simulink model "VCMGCM1962020b_v2"  (R2020b)
settings: Solver=FixedStepDiscrete  StartTime=0.0  StopTime=10.0  FixedStep=0.005  RelTol=1e-3  EnableMultiTasking=on
PreLoadFcn:
  | try, model_open; catch, disp('Error occurred while executing model pre-load callback: model_open.m'); disp('Please assure that the MATLAB working directory is set to the model directory before opening.'); end
InitFcn:
  | try, model_open; catch, end
undefined symbols (not defined in the file): Bridge, GCM, H, raptor_get_param_eval, raptor_get_safe_string, raptor_xcp_function
libraries: Blocks_lib x1165, Raptor_lib x665, simulink x62, VCM_lib x5
(part 16 of 23)

== system VCMGCM1962020b_v2/Fgnd/Actuators/CAN/Display/DisplayHVES1_D2/MsgTx ==
  Data : Inport
  Enable : EnablePort
  Bus Selector1 : BusSelector  OutputSignals=VirtualSensors.Batt.BattSOC [%]
  Bus Selector2 : BusSelector  OutputSignals=Sensors.CAN.Other.BCM.CCVS1_BCM.Parking_Brak_Switch.Parking_Brak_Switch [enum],VirtualSensors.Spd.VehSpd [kph]
  Bus Selector3 : BusSelector  OutputSignals=Sensors.CAN.Other.BCM.BCMAMB.Amb_Air_Temp.Amb_Air_Temp [C]
  Bus Selector4 : BusSelector  OutputSignals=VirtualSensors.Spd.VehOdmtr [km],VirtualSensors.Spd.TripDist [km]
  Bus Selector5 : BusSelector  OutputSignals=VirtualSensors.Batt.BattCur [A],VirtualSensors.Batt.BattVolt [V]
  Bus Selector6 : BusSelector  OutputSignals=Control.Other.Other.Regenstate
  Bus Selector7 : BusSelector  OutputSignals=Control.Mode.StartStop.ChgMode [Bool]
  Bus Selector8 : BusSelector  OutputSignals=VirtualSensors.Spd.VehRangeEst [km]
  Bus Selector9 : BusSelector  OutputSignals=Control.Mode.PRNDMode_Act [enum]
  CANTxField{,4..6,8..10} (7 alike) : Blocks_lib/CANTxField  Commented=on  custom=on  custom_nam=[nam '---']  custom_units='---'
  CANTxField{1..3,7} (4 alike) : Blocks_lib/CANTxField  custom=on  custom_nam=[nam '---']  custom_units='---'
  Header : Blocks_lib/Header  width=Landscape  addtext=''
  raptor_can_txmsg : Raptor_lib/CAN/raptor_can_txmsg  Commented=on  canDefinition=struct('dbcFile', 'Drivers_Disp_dbc_file_v5.0.dbc','message', 'CCVS1','comment', '','signals', {{'P_Brake_Switch','Whl_Veh_Spd'}},'enabled', [ 1 1;],'scaled', [ 1 1;],'canBus', 'bus','messageID', [ 419361263;],'idMask', [ 536870911;],'payloadMask', [],'payloadValue', [],'period', [ 100;],'mailbox', '''''','queueSize', [ 1;],'label', [ 1;],'ver', [ 2;],'showID', [ 0;],'showRaw', [ 0;],'fill', [ 0;],'editID', [ 0;],'signalOrder', [ 1;],'signalAscDes', [ 1;])  canBus=bus  queueSize=1  payloadMask=[]  payloadValue=[]  period=100  showID=0  label=1  idMask=hex2dec('1FFFFFFF')  fill=0  id=419361263  showRaw=0  signalOrder=1  signalInfo={{struct('Name', 'Whl_Veh_Spd','Startbit', [ 0;],'SignalSize', [ 16;],'ByteOrder', 'LittleEndian','ValueType', 'UNSIGNED','Class', 'uint16','Signed', [ 0;],'Factor', [ 0.0039063;],'Offset', [ 0;],'Min', [ 0;],'Max', [ 250.996;],'Units', 'Km/h','Comment', '','StartBit', [ 8;]),struct('Name', 'P_Brake_Switch','Startbit', [ 0;],'SignalSize', [ 2;],'ByteOrder', 'LittleEndian','ValueType', 'UNSIGNED','Class', 'uint8','Signed', [ 0;],'Factor', [ 1;],'Offset', [ 0;],'Min', [ 0;],'Max', [ 3;],'Units', 'enum','Comment', '','StartBit', [ 2;])}}
      settings: SourceProductName=Raptor
  raptor_can_txmsg1 : Raptor_lib/CAN/raptor_can_txmsg  canDefinition=struct('dbcFile', 'Drivers_Disp_dbc_file_v5.0.dbc','message', 'HVES1_D2','comment', '','signals', {{'Batt_SOC'}},'enabled', [ 1;],'scaled', [ 1;],'canBus', 'bus','messageID', [ 418419183;],'idMask', [ 536870911;],'payloadMask', [],'payloadValue', [],'period', [ 100;],'mailbox', '''''','queueSize', [ 1;],'label', [ 1;],'ver', [ 2;],'showID', [ 0;],'showRaw', [ 0;],'fill', [ 0;],'editID', [ 0;],'signalOrder', [ 1;],'signalAscDes', [ 1;])  canBus=bus  queueSize=1  payloadMask=[]  payloadValue=[]  period=100  showID=0  label=1  idMask=hex2dec('1FFFFFFF')  fill=0  id=418419183  showRaw=0  signalOrder=1  signalInfo={{struct('Name', 'Batt_SOC','Startbit', [ 0;],'SignalSize', [ 16;],'ByteOrder', 'LittleEndian','ValueType', 'UNSIGNED','Class', 'uint16','Signed', [ 0;],'Factor', [ 0.0015625;],'Offset', [ 0;],'Min', [ 0;],'Max', [ 100.398;],'Units', '%','Comment', '','StartBit', [ 0;])}}
      settings: SourceProductName=Raptor
  raptor_can_txmsg2 : Raptor_lib/CAN/raptor_can_txmsg  Commented=on  canDefinition=struct('dbcFile', 'Drivers_Disp_dbc_file_v5.0.dbc','message', 'AMB','comment', '','signals', {{'Ambient_Air_Temperature','Cab_Temp'}},'enabled', [ 1 0;],'scaled', [ 1 1;],'canBus', 'bus','messageID', [ 419362081;],'idMask', [ 536870911;],'payloadMask', [],'payloadValue', [],'period', [ 100;],'mailbox', '''''','queueSize', [ 1;],'label', [ 1;],'ver', [ 2;],'showID', [ 0;],'showRaw', [ 0;],'fill', [ 0;],'editID', [ 0;],'signalOrder', [ 1;],'signalAscDes', [ 1;])  canBus=bus  queueSize=1  payloadMask=[]  payloadValue=[]  period=100  showID=0  label=1  idMask=hex2dec('1FFFFFFF')  fill=0  id=419362081  showRaw=0  signalOrder=1  signalInfo={{struct('Name', 'Ambient_Air_Temperature','Startbit', [ 0;],'SignalSize', [ 16;],'ByteOrder', 'LittleEndian','ValueType', 'UNSIGNED','Class', 'uint16','Signed', [ 0;],'Factor', [ 0.03125;],'Offset', [ -22;],'Min', [ -22;],'Max', [ 140;],'Units', 'C','Comment', '','StartBit', [ 24;]),struct('Name', 'Cab_Temp','Startbit', [ 0;],'SignalSize', [ 16;],'ByteOrder', 'LittleEndian','ValueType', 'UNSIGNED','Class', 'uint16','Signed', [ 0;],'Factor', [ 0.03125;],'Offset', [ -22;],'Min', [ -22;],'Max', [ 140;],'Units', 'C','Comment', '','StartBit', [ 8;])}}
      settings: SourceProductName=Raptor
  raptor_can_txmsg3 : Raptor_lib/CAN/raptor_can_txmsg  canDefinition=struct('dbcFile', 'Drivers_Disp_dbc_file_v5.0.dbc','message', 'OI','comment', '','signals', {{'Range_Estimate'}},'enabled', [ 1;],'scaled', [ 1;],'canBus', 'bus','messageID', [ 419364847;],'idMask', [ 536870911;],'payloadMask', [],'payloadValue', [],'period', [ 100;],'mailbox', '''''','queueSize', [ 1;],'label', [ 1;],'ver', [ 2;],'showID', [ 0;],'showRaw', [ 0;],'fill', [ 0;],'editID', [ 0;],'signalOrder', [ 1;],'signalAscDes', [ 1;])  canBus=bus  queueSize=1  payloadMask=[]  payloadValue=[]  period=100  showID=0  label=1  idMask=hex2dec('1FFFFFFF')  fill=0  id=419364847  showRaw=0  signalOrder=1  signalInfo={{struct('Name', 'Range_Estimate','Startbit', [ 0;],'SignalSize', [ 16;],'ByteOrder', 'LittleEndian','ValueType', 'UNSIGNED','Class', 'uint16','Signed', [ 0;],'Factor', [ 1;],'Offset', [ 0;],'Min', [ 0;],'Max', [ 64255;],'Units', 'km','Comment', '','StartBit', [ 16;])}}
      settings: SourceProductName=Raptor
  raptor_can_txmsg4 : Raptor_lib/CAN/raptor_can_txmsg  canDefinition=struct('dbcFile', 'Drivers_Disp_dbc_file_v5.0.dbc','message', 'VDHR','comment', '','signals', {{'Tot_Veh_Dist','Trip_Dist'}},'enabled', [ 1 1;],'scaled', [ 1 1;],'canBus', 'bus','messageID', [ 419348975;],'idMask', [ 536870911;],'payloadMask', [],'payloadValue', [],'period', [ 100;],'mailbox', '''''','queueSize', [ 1;],'label', [ 1;],'ver', [ 2;],'showID', [ 0;],'showRaw', [ 0;],'fill', [ 0;],'editID', [ 0;],'signalOrder', [ 1;],'signalAscDes', [ 1;])  canBus=bus  queueSize=1  payloadMask=[]  payloadValue=[]  period=100  showID=0  label=1  idMask=hex2dec('1FFFFFFF')  fill=0  id=419348975  showRaw=0  signalOrder=1  signalInfo={{struct('Name', 'Tot_Veh_Dist','Startbit', [ 0;],'SignalSize', [ 32;],'ByteOrder', 'LittleEndian','ValueType', 'UNSIGNED','Class', 'uint32','Signed', [ 0;],'Factor', [ 5;],'Offset', [ 0;],'Min', [ 0;],'Max', [ 419436000;],'Units', 'm','Comment', '','StartBit', [ 0;]),struct('Name', 'Trip_Dist','Startbit', [ 0;],'SignalSize', [ 32;],'ByteOrder', 'LittleEndian','ValueType', 'UNSIGNED','Class', 'uint32','Signed', [ 0;],'Factor', [ 5;],'Offset', [ 0;],'Min', [ 0;],'Max', [ 419436000;],'Units', 'm','Comment', '','StartBit', [ 32;])}}
      settings: SourceProductName=Raptor
  raptor_can_txmsg5 : Raptor_lib/CAN/raptor_can_txmsg  Commented=on  canDefinition=struct('dbcFile', 'Drivers_Disp_dbc_file_v3.dbc','message', 'HVES1_D1','comment', '','signals', {{'Batt_Current','Batt_Voltage_Level'}},'enabled', [ 1 1;],'scaled', [ 1 1;],'canBus', 'bus','messageID', [ 217092335;],'idMask', [ 536870911;],'payloadMask', [],'payloadValue', [],'period', [ 100;],'mailbox', '''''','queueSize', [ 1;],'label', [ 1;],'ver', [ 2;],'showID', [ 0;],'showRaw', [ 0;],'fill', [ 0;],'editID', [ 0;],'signalOrder', [ 1;],'signalAscDes', [ 1;])  canBus=bus  queueSize=1  payloadMask=[]  payloadValue=[]  period=100  showID=0  label=1  idMask=hex2dec('1FFFFFFF')  fill=0  id=217092335  showRaw=0  signalOrder=1  signalInfo={{struct('Name', 'Batt_Voltage_Level','Startbit', [ 0;],'SignalSize', [ 16;],'ByteOrder', 'LittleEndian','ValueType', 'UNSIGNED','Class', 'uint16','Signed', [ 0;],'Factor', [ 0.05;],'Offset', [ 0;],'Min', [ 0;],'Max', [ 3212.75;],'Units', 'V','Comment', '','StartBit', [ 32;]),struct('Name', 'Batt_Current','Startbit', [ 0;],'SignalSize', [ 16;],'ByteOrder', 'LittleEndian','ValueType', 'UNSIGNED','Class', 'uint16','Signed', [ 0;],'Factor', [ 0.05;],'Offset', [ -1600;],'Min', [ -1600;],'Max', [ 1612.75;],'Units', 'A','Comment', '','StartBit', [ 48;])}}
      settings: SourceProductName=Raptor
  raptor_can_txmsg6 : Raptor_lib/CAN/raptor_can_txmsg  canDefinition=struct('dbcFile', 'Drivers_Disp_dbc_file_v5.0.dbc','message', 'HSS1','comment', '','signals', {{'Regen_Braking_Indicator'}},'enabled', [ 1;],'scaled', [ 1;],'canBus', 'bus','messageID', [ 419218159;],'idMask', [ 536870911;],'payloadMask', [],'payloadValue', [],'period', [ 100;],'mailbox', '''''','queueSize', [ 1;],'label', [ 1;],'ver', [ 2;],'showID', [ 0;],'showRaw', [ 0;],'fill', [ 0;],'editID', [ 0;],'signalOrder', [ 1;],'signalAscDes', [ 1;])  canBus=bus  queueSize=1  payloadMask=[]  payloadValue=[]  period=100  showID=0  label=1  idMask=hex2dec('1FFFFFFF')  fill=0  id=419218159  showRaw=0  signalOrder=1  signalInfo={{struct('Name', 'Regen_Braking_Indicator','Startbit', [ 0;],'SignalSize', [ 2;],'ByteOrder', 'LittleEndian','ValueType', 'UNSIGNED','Class', 'uint8','Signed', [ 0;],'Factor', [ 1;],'Offset', [ 0;],'Min', [ 0;],'Max', [ 3;],'Units', 'enum','Comment', '','StartBit', [ 20;])}}
      settings: SourceProductName=Raptor
  raptor_can_txmsg7 : Raptor_lib/CAN/raptor_can_txmsg  Commented=on  canDefinition=struct('dbcFile', 'Drivers_Disp_dbc_file_v3.dbc','message', 'BCH1','comment', '','signals', {{'Batt_Charger1_State','Batt_Charger_Output_Curr','Batt_Charger_Output_Volt'}},'enabled', [ 1 0 0;],'scaled', [ 1 1 1;],'canBus', 'bus','messageID', [ 419239407;],'idMask', [ 536870911;],'payloadMask', [],'payloadValue', [],'period', [ 100;],'mailbox', '''''','queueSize', [ 1;],'label', [ 1;],'ver', [ 2;],'showID', [ 0;],'showRaw', [ 0;],'fill', [ 0;],'editID', [ 0;],'signalOrder', [ 1;],'signalAscDes', [ 1;])  canBus=bus  queueSize=1  payloadMask=[]  payloadValue=[]  period=100  showID=0  label=1  idMask=hex2dec('1FFFFFFF')  fill=0  id=419239407  showRaw=0  signalOrder=1  signalInfo={{struct('Name', 'Batt_Charger1_State','Startbit', [ 0;],'SignalSize', [ 4;],'ByteOrder', 'LittleEndian','ValueType', 'UNSIGNED','Class', 'uint8','Signed', [ 0;],'Factor', [ 1;],'Offset', [ 0;],'Min', [ 0;],'Max', [ 15;],'Units', 'enum','Comment', '','StartBit', [ 0;]),struct('Name', 'Batt_Charger_Output_Volt','Startbit', [ 0;],'SignalSize', [ 16;],'ByteOrder', 'LittleEndian','ValueType', 'UNSIGNED','Class', 'uint16','Signed', [ 0;],'Factor', [ 0.05;],'Offset', [ 0;],'Min', [ 0;],'Max', [ 3212.75;],'Units', 'V','Comment', '','StartBit', [ 8;]),struct('Name', 'Batt_Charger_Output_Curr','Startbit', [ 0;],'SignalSize', [ 16;],'ByteOrder', 'LittleEndian','ValueType', 'UNSIGNED','Class', 'uint16','Signed', [ 0;],'Factor', [ 0.05;],'Offset', [ -1600;],'Min', [ -1600;],'Max', [ 1612.75;],'Units', 'A','Comment', '','StartBit', [ 24;])}}
      settings: SourceProductName=Raptor
  raptor_can_txmsg8 : Raptor_lib/CAN/raptor_can_txmsg  Commented=on  canDefinition=struct('dbcFile', 'Drivers_Disp_dbc_file_v3.dbc','message', 'ETC2','comment', '','signals', {{'Transmssn_Curr_Gear'}},'enabled', [ 1;],'scaled', [ 1;],'canBus', 'bus','messageID', [ 418383343;],'idMask', [ 536870911;],'payloadMask', [],'payloadValue', [],'period', [ 100;],'mailbox', '''''','queueSize', [ 1;],'label', [ 1;],'ver', [ 2;],'showID', [ 0;],'showRaw', [ 0;],'fill', [ 0;],'editID', [ 0;],'signalOrder', [ 1;],'signalAscDes', [ 1;])  canBus=bus  queueSize=1  payloadMask=[]  payloadValue=[]  period=100  showID=0  label=1  idMask=hex2dec('1FFFFFFF')  fill=0  id=418383343  showRaw=0  signalOrder=1  signalInfo={{struct('Name', 'Transmssn_Curr_Gear','Startbit', [ 0;],'SignalSize', [ 8;],'ByteOrder', 'LittleEndian','ValueType', 'UNSIGNED','Class', 'uint8','Signed', [ 0;],'Factor', [ 1;],'Offset', [ 0;],'Min', [ -125;],'Max', [ 125;],'Units', 'gear','Comment', '','StartBit', [ 32;])}}
      settings: SourceProductName=Raptor
  wires:
  CANTxField/1 -> raptor_can_txmsg/1  "P_Brake_Switch"
  Bus Selector2/1 -> CANTxField/1  "<Parking_Brak_Switch [enum]>"
  CANTxField3/1 -> raptor_can_txmsg1/1  "Batt_SOC"
  Bus Selector1/1 -> CANTxField3/1  "<BattSOC [%]>"
  Bus Selector3/1 -> CANTxField4/1  "<Amb_Air_Temp [C]>"
  CANTxField4/1 -> raptor_can_txmsg2/1  "Ambient_Air_Temperature"
  CANTxField1/1 -> raptor_can_txmsg3/1  "Range_Estimate"
  Bus Selector8/1 -> CANTxField1/1  "<VehRangeEst [km]>"
  CANTxField2/1 -> raptor_can_txmsg4/1  "Tot_Veh_Dist"
  Bus Selector4/1 -> CANTxField2/1  "<VehOdmtr [km]>"
  Bus Selector5/1 -> CANTxField5/1  "<BattCur [A]>"
  CANTxField5/1 -> raptor_can_txmsg5/1  "Batt_Current"
  Bus Selector5/2 -> CANTxField6/1  "<BattVolt [V]>"
  CANTxField6/1 -> raptor_can_txmsg5/2  "Batt_Voltage_Level"
  Bus Selector6/1 -> CANTxField7/1  "<Regenstate>"
  CANTxField7/1 -> raptor_can_txmsg6/1  "Regen_Braking_Indicator"
  CANTxField8/1 -> raptor_can_txmsg7/1  "Batt_Charger1_State"
  Bus Selector7/1 -> CANTxField8/1  "<ChgMode [Bool]>"
  Data/1 -> Bus Selector8/1, Bus Selector9/1, Bus Selector7/1, Bus Selector6/1, Bus Selector5/1, Bus Selector4/1, Bus Selector3/1, Bus Selector1/1, Bus Selector2/1
  Bus Selector4/2 -> raptor_can_txmsg4/2  "<TripDist [km]>"
  Bus Selector9/1 -> CANTxField9/1  "<PRNDMode_Act [enum]>"
  CANTxField9/1 -> raptor_can_txmsg8/1  "Transmssn_Curr_Gear"
  Bus Selector2/2 -> CANTxField10/1  "<VehSpd [kph]>"
  CANTxField10/1 -> raptor_can_txmsg/2  "Whl_Veh_Spd"

== system VCMGCM1962020b_v2/Fgnd/Actuators/CAN/Drive Inverter/DrvInvtrNMT/MsgTx ==
  State : Inport
  Trigger : TriggerPort  VariantControl=(inherit)  PortDimensions=1
  Bus Selector : BusSelector  OutputSignals=NMT_State,NMT_Trg
  Header : Blocks_lib/Header  width=Landscape  addtext=''
  raptor_can_txmsg : Raptor_lib/CAN/raptor_can_txmsg  canDefinition=struct('dbcFile', '20220526e_emDrive_NodeID_0x01.dbc','message', 'NMT','comment', 'CANopen Network management message','signals', {{'NMT_StateDmd','NMT_TargetNode'}},'enabled', [ 1 1;],'scaled', [ 1 1;],'canBus', '''CAN3''','messageID', [ 0;],'idMask', [ 536870911;],'payloadMask', [],'payloadValue', [],'period', [ -1;],'mailbox', '','queueSize', [ 1;],'label', [ 0;],'ver', [ 2;],'showID', [ 0;],'showRaw', [ 0;],'fill', [ 0;],'editID', [ 0;],'signalOrder', [ 1;],'signalAscDes', [ 1;])  canBus='CAN3'  queueSize=1  payloadMask=[]  payloadValue=[]  period=-1  showID=0  label=0  idMask=hex2dec('1FFFFFFF')  fill=0  id=0  showRaw=0  signalOrder=1  signalInfo={{struct('Name', 'NMT_StateDmd','Startbit', [ 0;],'SignalSize', [ 8;],'ByteOrder', 'LittleEndian','ValueType', 'UNSIGNED','Class', 'uint8','Signed', [ 0;],'Factor', [ 1;],'Offset', [ 0;],'Min', [ 0;],'Max', [ 0;],'Units', '','Comment', '','StartBit', [ 0;]),struct('Name', 'NMT_TargetNode','Startbit', [ 0;],'SignalSize', [ 8;],'ByteOrder', 'LittleEndian','ValueType', 'UNSIGNED','Class', 'uint8','Signed', [ 0;],'Factor', [ 1;],'Offset', [ 0;],'Min', [ 0;],'Max', [ 127;],'Units', '','Comment', '','StartBit', [ 8;])}}
      settings: SourceProductName=Raptor
  wires:
  State/1 -> Bus Selector/1
  Bus Selector/2 -> raptor_can_txmsg/2  "<NMT_Trg>"
  Bus Selector/1 -> raptor_can_txmsg/1  "<NMT_State>"

== system VCMGCM1962020b_v2/Fgnd/Actuators/CAN/Drive Inverter/DrvInvtrVCU1/MsgTx ==
  State : Inport
  Enable : EnablePort
  Bus Selector1 : BusSelector  OutputSignals=VCUStateCMD
  CANTxField : Blocks_lib/CANTxField  custom=on  custom_nam=[nam '---']  custom_units='---'
  Header : Blocks_lib/Header  width=Landscape  addtext=''
  raptor_can_txmsg : Raptor_lib/CAN/raptor_can_txmsg  canDefinition=struct('dbcFile', '20220526e_emDrive_NodeID_0x01.dbc','message', 'VCU1','comment', '100-200ms. Timeout 250ms','signals', {{'VCU1_StateCmd','VCU_TrqLim'}},'enabled', [ 1 0;],'scaled', [ 1 1;],'canBus', '''CAN3''','messageID', [ 513;],'idMask', [ 536870911;],'payloadMask', [],'payloadValue', [],'period', [ 50;],'mailbox', '','queueSize', [ 1;],'label', [ 0;],'ver', [ 2;],'showID', [ 0;],'showRaw', [ 0;],'fill', [ 0;],'editID', [ 0;],'signalOrder', [ 1;],'signalAscDes', [ 1;])  canBus='CAN3'  queueSize=1  payloadMask=[]  payloadValue=[]  period=50  showID=0  label=0  idMask=hex2dec('1FFFFFFF')  fill=0  id=513  showRaw=0  signalOrder=1  signalInfo={{struct('Name', 'VCU1_StateCmd','Startbit', [ 0;],'SignalSize', [ 8;],'ByteOrder', 'LittleEndian','ValueType', 'UNSIGNED','Class', 'uint8','Signed', [ 0;],'Factor', [ 1;],'Offset', [ 0;],'Min', [ 0;],'Max', [ 2;],'Units', 'enum','Comment', 'Application_Control__Control','StartBit', [ 0;]),struct('Name', 'VCU_TrqLim','Startbit', [ 0;],'SignalSize', [ 8;],'ByteOrder', 'LittleEndian','ValueType', 'UNSIGNED','Class', 'uint8','Signed', [ 0;],'Factor', [ 1;],'Offset', [ 0;],'Min', [ 0;],'Max', [ 255;],'Units', 'Nm','Comment', 'Motor Torque Limit defined by VCU','StartBit', [ 8;])}}
      settings: SourceProductName=Raptor
  wires:
  CANTxField/1 -> raptor_can_txmsg/1  "VCU1_StateCmd"
  State/1 -> Bus Selector1/1
  Bus Selector1/1 -> CANTxField/1  "<VCUStateCMD>"

== system VCMGCM1962020b_v2/Fgnd/Actuators/CAN/Drive Inverter/DrvInvtrVCU2/MsgTx ==
  State : Inport
  Enable : EnablePort
  Bus Selector : BusSelector  OutputSignals=StateTrqCmd,StateSpdCmd
  Header : Blocks_lib/Header  width=Landscape  addtext=''
  raptor_can_txmsg : Raptor_lib/CAN/raptor_can_txmsg  canDefinition=struct('dbcFile', '20220526e_emDrive_NodeID_0x01.dbc','message', 'VCU2','comment', '20-50ms. Timeout 100ms','signals', {{'VCU2_EmTorqDmd','VCU2_EmVelDmd'}},'enabled', [ 1 1;],'scaled', [ 1 1;],'canBus', '''CAN3''','messageID', [ 769;],'idMask', [ 536870911;],'payloadMask', [],'payloadValue', [],'period', [ 50;],'mailbox', '','queueSize', [ 1;],'label', [ 0;],'ver', [ 2;],'showID', [ 0;],'showRaw', [ 0;],'fill', [ 0;],'editID', [ 0;],'signalOrder', [ 1;],'signalAscDes', [ 1;])  canBus='CAN3'  queueSize=1  payloadMask=[]  payloadValue=[]  period=50  showID=0  label=0  idMask=hex2dec('1FFFFFFF')  fill=0  id=769  showRaw=0  signalOrder=1  signalInfo={{struct('Name', 'VCU2_EmTorqDmd','Startbit', [ 0;],'SignalSize', [ 32;],'ByteOrder', 'LittleEndian','ValueType', 'FLOAT32','Class', 'single','Signed', [ 1;],'Factor', [ 1;],'Offset', [ 0;],'Min', [ -200;],'Max', [ 200;],'Units', 'Nm','Comment', 'Application_Control__TorqueRef','StartBit', [ 0;]),struct('Name', 'VCU2_EmVelDmd','Startbit', [ 0;],'SignalSize', [ 32;],'ByteOrder', 'LittleEndian','ValueType', 'FLOAT32','Class', 'single','Signed', [ 1;],'Factor', [ 1;],'Offset', [ 0;],'Min', [ -10000;],'Max', [ 10000;],'Units', 'rpm','Comment', 'Application_Control__VelocityRef','StartBit', [ 32;])}}
      settings: SourceProductName=Raptor
  wires:
  State/1 -> Bus Selector/1
  Bus Selector/1 -> raptor_can_txmsg/1  "<StateTrqCmd>"
  Bus Selector/2 -> raptor_can_txmsg/2  "<StateSpdCmd>"

== system VCMGCM1962020b_v2/Fgnd/Actuators/CAN/Drive Inverter/Function-Call Subsystem/MsgName ==
  Constant : Constant  Value=uint8(3)
  Constant1 : Constant  Value=uint8(1)
  Header1 : Blocks_lib/Header  width=Landscape  addtext=''
  raptor_can_txmsg : Raptor_lib/CAN/raptor_can_txmsg  canDefinition=struct('dbcFile', '20220526e_emDrive_NodeID_0x01.dbc','message', 'NMT','comment', 'CANopen Network management message','signals', {{'NMT_StateDmd','NMT_TargetNode'}},'enabled', [ 1 1;],'scaled', [ 1 1;],'canBus', '''CAN1''','messageID', [ 0;],'idMask', [ 536870911;],'payloadMask', [],'payloadValue', [],'period', [ 0;],'mailbox', '','queueSize', [ 1;],'label', [ 0;],'ver', [ 2;],'showID', [ 0;],'showRaw', [ 0;],'showRawMsg', [ 0;],'fill', [ 0;],'editID', [ 0;],'signalOrder', [ 1;],'signalAscDes', [ 1;])  canBus='CAN1'  queueSize=1  payloadMask=[]  payloadValue=[]  period=0  showID=0  label=0  idMask=hex2dec('1FFFFFFF')  fill=0  id=0  showRaw=0  signalOrder=1  signalInfo={{struct('Name', 'NMT_StateDmd','Startbit', [ 0;],'SignalSize', [ 8;],'ByteOrder', 'LittleEndian','ValueType', 'UNSIGNED','Class', 'uint8','Signed', [ 0;],'Factor', [ 1;],'Offset', [ 0;],'Min', [ 0;],'Max', [ 0;],'Units', '','Comment', '','StartBit', [ 0;]),struct('Name', 'NMT_TargetNode','Startbit', [ 0;],'SignalSize', [ 8;],'ByteOrder', 'LittleEndian','ValueType', 'UNSIGNED','Class', 'uint8','Signed', [ 0;],'Factor', [ 1;],'Offset', [ 0;],'Min', [ 0;],'Max', [ 127;],'Units', '','Comment', '','StartBit', [ 8;])}}
      settings: SourceProductName=Raptor
  wires:
  Constant/1 -> raptor_can_txmsg/1  "NMT_StateDmd"
  Constant1/1 -> raptor_can_txmsg/2  "NMT_TargetNode"

== system VCMGCM1962020b_v2/Fgnd/Actuators/CAN/Drive Inverter/NMT Trasition Command/Error ==
  Action Port : ActionPort  ActionPortLabel=case [ 6 ]:
  Bus Creator : BusCreator  Inputs=7
  Constant1 : Constant  Value=double(0)
  Constant2 : Constant  Value=boolean(1)
  Constant3 : Constant  Value=double(0)
  Constant4 : Constant  Value=boolean(0)
  Constant5 : Constant  Value=uint8(0)
  Constant6 : Constant  Value=uint8(0)
  Constant7 : Constant  Value=uint8(2)
  Header : Blocks_lib/Header  width=Portrait  addtext=''
  Cmd : Outport  VectorParamsAs1DForOutWhenUnconnected=off
  wires:
  Constant4/1 -> Bus Creator/5  "NMT_Xmit [bool]"
  Constant5/1 -> Bus Creator/6  "NMT_StateDmd"
  Constant3/1 -> Bus Creator/2  "TrqCmd [Nm]"
  Constant1/1 -> Bus Creator/3  "SpdCmd [rpm]"
  Constant2/1 -> Bus Creator/4  "VCU1_2_Transmit [bool]"
  Constant6/1 -> Bus Creator/7  "NMT_Target_Node"
  Bus Creator/1 -> Cmd/1
  Constant7/1 -> Bus Creator/1  "VCU1StateCmd [bool]"

== system VCMGCM1962020b_v2/Fgnd/Actuators/CAN/Drive Inverter/NMT Trasition Command/Error1 ==
  Action Port : ActionPort  ActionPortLabel=case [ 7 ]:
  Bus Creator : BusCreator  Inputs=7
  Constant1 : Constant  Value=double(0)
  Constant2 : Constant  Value=boolean(1)
  Constant3 : Constant  Value=double(0)
  Constant4 : Constant  Value=boolean(1)
  Constant5 : Constant  Value=uint8(2)
  Constant6 : Constant  Value=uint8(1)
  Constant7 : Constant  Value=uint8(0)
  Header : Blocks_lib/Header  width=Portrait  addtext=''
  Cmd : Outport  VectorParamsAs1DForOutWhenUnconnected=off
  wires:
  Constant4/1 -> Bus Creator/5  "NMT_Xmit [bool]"
  Constant5/1 -> Bus Creator/6  "NMT_StateDmd"
  Constant3/1 -> Bus Creator/2  "TrqCmd [Nm]"
  Constant1/1 -> Bus Creator/3  "SpdCmd [rpm]"
  Constant2/1 -> Bus Creator/4  "VCU1_2_Transmit [bool]"
  Constant6/1 -> Bus Creator/7  "NMT_Target_Node"
  Bus Creator/1 -> Cmd/1
  Constant7/1 -> Bus Creator/1  "VCU1StateCmd [bool]"

== system VCMGCM1962020b_v2/Fgnd/Actuators/CAN/Drive Inverter/NMT Trasition Command/Error2 ==
  Action Port : ActionPort  ActionPortLabel=case [ 10 ]:
  Bus Creator : BusCreator  Inputs=7
  Constant1 : Constant  Value=double(0)
  Constant2 : Constant  Value=boolean(1)
  Constant3 : Constant  Value=double(0)
  Constant4 : Constant  Value=boolean(1)
  Constant5 : Constant  Value=uint8(2)
  Constant6 : Constant  Value=uint8(1)
  Constant7 : Constant  Value=uint8(2)
  Header : Blocks_lib/Header  width=Portrait  addtext=''
  Cmd : Outport  VectorParamsAs1DForOutWhenUnconnected=off
  wires:
  Constant4/1 -> Bus Creator/5  "NMT_Xmit [bool]"
  Constant5/1 -> Bus Creator/6  "NMT_StateDmd"
  Constant3/1 -> Bus Creator/2  "TrqCmd [Nm]"
  Constant1/1 -> Bus Creator/3  "SpdCmd [rpm]"
  Constant2/1 -> Bus Creator/4  "VCU1_2_Transmit [bool]"
  Constant6/1 -> Bus Creator/7  "NMT_Target_Node"
  Bus Creator/1 -> Cmd/1
  Constant7/1 -> Bus Creator/1  "VCU1StateCmd [bool]"

== system VCMGCM1962020b_v2/Fgnd/Actuators/CAN/Drive Inverter/NMT Trasition Command/Init State ==
  Action Port : ActionPort  ActionPortLabel=case [ 3 ]:
  Bus Creator : BusCreator  Inputs=7
  Constant1 : Constant  Value=double(0)
  Constant2 : Constant  Value=boolean(1)
  Constant3 : Constant  Value=double(0)
  Constant4 : Constant  Value=boolean(0)
  Constant5 : Constant  Value=uint8(0)
  Constant6 : Constant  Value=uint8(0)
  Constant7 : Constant  Value=uint8(0)
  Header : Blocks_lib/Header  width=Portrait  addtext=''
  Cmd : Outport  VectorParamsAs1DForOutWhenUnconnected=off
  wires:
  Constant6/1 -> Bus Creator/7  "NMT_Target_Node"
  Constant2/1 -> Bus Creator/4  "VCU1_2_Transmit [bool]"
  Bus Creator/1 -> Cmd/1
  Constant4/1 -> Bus Creator/5  "NMT_Xmit [bool]"
  Constant1/1 -> Bus Creator/3  "SpdCmd [rpm]"
  Constant3/1 -> Bus Creator/2  "TrqCmd [Nm]"
  Constant5/1 -> Bus Creator/6  "NMT_StateDmd"
  Constant7/1 -> Bus Creator/1  "VCU1StateCmd [bool]"

== system VCMGCM1962020b_v2/Fgnd/Actuators/CAN/Drive Inverter/NMT Trasition Command/Inverter Error Reset ==
  note: This logic forces an inverter error reset during transition from of to Runmode. Used during development
  Data : Inport
  StateCmd : Inport  Port=2
  Bus Selector2 : BusSelector  OutputSignals=Control.DrvInvtr.DrvInvtrEnblReq [Bool]
  CntrSat1 : Blocks_lib/CntrSat  init=0  inc=1  typ=uint8  relop=>=  th_nam='InvrteOffDwll'  th_gain=samptime  th_units='sec'  th_help='Dwell time to send inverter off command during startup'  th_group='Group'
  CntrSat2 : Blocks_lib/CntrSat  init=0  inc=1  typ=uint8  relop=>=  th_nam='InvrteErrRstDwll'  th_gain=samptime  th_units='sec'  th_help='Dwelltime to time to send Invtr error reset'  th_group='Group'
  Data Type Conversion : DataTypeConversion  OutDataTypeStr=uint8
  Err_Reset : Constant  Value=2  OutDataTypeStr=uint8
  Header : Blocks_lib/Header  width=Landscape  addtext=''
  Off : Constant  Value=0  OutDataTypeStr=uint8
  Off1 : Constant  Value=0  OutDataTypeStr=uint8
  SetRst : Blocks_lib/SetRst  init=0
  Switch{,1..3} (4 alike) : Switch  Criteria=u2 > Threshold
  raptor_adjustment : Raptor_lib/Data Storage/raptor_adjustment  paramName='InvrtrForceErrRst'  nameSource=Parameter  initValue=1  dataType=boolean  storage=Calibration  calDispType=Number  calEnum={'False', 'True'}  calGain=1.0  calOffset=0.0  calMax=inf  calMin=-inf  calFormat='-1'  calUnit='Bool'  calHelp='This will force the inverter to clear errors and restart at RunMode'  calAccess=1  calFunction=' Actuators | Inverter'  calDispHeaders=off  calColHeaders={'Col1' 'Col2' 'Col3'}  calRowHeaders={'Row1' 'Row2' 'Row3'}
      settings: SourceProductName=Raptor
  raptor_measurement1 : Raptor_lib/Data Storage/raptor_measurement  paramName='Test_Var1'  nameSource=Parameter  calDispType=Number  calEnum={'Disabled', 'Enabled'}  calGain=1  calOffset=0  calMax=inf  calMin=-inf  calFormat=''  calUnit='uint8'  calHelp='Test Variable'  calAccess=1  calFunction=' Actuator | Test'  calVisible=on
      settings: SourceProductName=Raptor
  raptor_measurement2 : Raptor_lib/Data Storage/raptor_measurement  paramName='Test_Var2'  nameSource=Parameter  calDispType=Number  calEnum={'Disabled', 'Enabled'}  calGain=1  calOffset=0  calMax=inf  calMin=-inf  calFormat=''  calUnit='uint8'  calHelp='Test Variable'  calAccess=1  calFunction=' Actuator | Test'  calVisible=on
      settings: SourceProductName=Raptor
  raptor_measurement3 : Raptor_lib/Data Storage/raptor_measurement  paramName='Test_Var3'  nameSource=Parameter  calDispType=Number  calEnum={'Disabled', 'Enabled'}  calGain=1  calOffset=0  calMax=inf  calMin=-inf  calFormat=''  calUnit='uint8'  calHelp='Test Variable'  calAccess=1  calFunction=' Actuator | Test'  calVisible=on
      settings: SourceProductName=Raptor
  rising edge2 : Subsystem
  InverterStateCmd : Outport
  wires:
  Bus Selector2/1 -> Switch3/2, rising edge2/1(<RunMode [Bool]>), raptor_measurement3/1, Data Type Conversion/1, CntrSat2/1  "<DrvInvtrEnblReq [Bool]>"
  CntrSat2/1 -> raptor_measurement1/1, CntrSat1/1, Switch/2
  Off/1 -> Switch/1
  rising edge2/1(rising) -> CntrSat1/2, SetRst/2, CntrSat2/2
  Switch/1 -> Switch1/3
  Data/1 -> Bus Selector2/1
  Switch2/1 -> InverterStateCmd/1
  Switch1/1 -> Switch2/1
  StateCmd/1 -> Switch2/3
  raptor_adjustment/1 -> Switch2/2
  CntrSat1/1 -> raptor_measurement2/1, SetRst/1
  Data Type Conversion/1 -> Switch1/1
  SetRst/1 -> Switch1/2
  Err_Reset/1 -> Switch3/1
  Switch3/1 -> Switch/3
  Off1/1 -> Switch3/3

== system VCMGCM1962020b_v2/Fgnd/Actuators/CAN/Drive Inverter/NMT Trasition Command/Off ==
  Action Port : ActionPort  ActionPortLabel=case [ 4 ]:
  Bus Creator : BusCreator  Inputs=7
  Constant1 : Constant  Value=double(0)
  Constant2 : Constant  Value=boolean(1)
  Constant3 : Constant  Value=double(0)
  Constant4 : Constant  Value=boolean(1)
  Constant5 : Constant  Value=uint8(1)
  Constant6 : Constant  Value=uint8(1)
  Constant7 : Constant  Value=uint8(0)
  Header : Blocks_lib/Header  width=Portrait  addtext=''
  Cmd : Outport  VectorParamsAs1DForOutWhenUnconnected=off
  wires:
  Constant4/1 -> Bus Creator/5  "NMT_Xmit [bool]"
  Constant5/1 -> Bus Creator/6  "NMT_StateDmd"
  Constant3/1 -> Bus Creator/2  "TrqCmd [Nm]"
  Constant1/1 -> Bus Creator/3  "SpdCmd [rpm]"
  Constant2/1 -> Bus Creator/4  "VCU1_2_Transmit [bool]"
  Constant6/1 -> Bus Creator/7  "NMT_Target_Node"
  Bus Creator/1 -> Cmd/1
  Constant7/1 -> Bus Creator/1  "VCU1StateCmd [bool]"

== system VCMGCM1962020b_v2/Fgnd/Actuators/CAN/Drive Inverter/NMT Trasition Command/Run ==
  Input : Inport
  Action Port : ActionPort  ActionPortLabel=case [ 5 ]:
  Bus Creator1 : BusCreator  Inputs=7
  Bus Selector1 : BusSelector  OutputSignals=Control.DrvInvtr.MtrTrqReq.DrvTrqReq.DrvTrqReqFinal [Nm]
  Constant10 : Constant  Value=uint8(1)
  Constant11 : Constant  Value=uint8(1)
  Constant3 : Constant  Value=double(0)
  Constant6 : Constant  Value=boolean(1)
  Constant8 : Constant  Value=boolean(0)
  Constant9 : Constant  Value=uint8(1)
  Header : Blocks_lib/Header  width=Portrait  addtext=''
  Zero-Order Hold : ZeroOrderHold  SampleTime=-1
  Cmd1 : Outport  VectorParamsAs1DForOutWhenUnconnected=off
  wires:
  Bus Selector1/1 -> Zero-Order Hold/1  "<DrvTrqReqFinal [Nm]>"
  Input/1 -> Bus Selector1/1
  Constant11/1 -> Bus Creator1/1  "VCU1StateCmd [bool]"
  Bus Creator1/1 -> Cmd1/1
  Constant3/1 -> Bus Creator1/3  "SpdCmd [rpm]"
  Zero-Order Hold/1 -> Bus Creator1/2  "TrqCmd [Nm]"
  Constant10/1 -> Bus Creator1/7  "NMT_Target_Node"
  Constant8/1 -> Bus Creator1/5  "NMT_Xmit [bool]"
  Constant9/1 -> Bus Creator1/6  "NMT_StateDmd"
  Constant6/1 -> Bus Creator1/4  "VCU1_2_Transmit [bool]"

== system VCMGCM1962020b_v2/Fgnd/Actuators/CAN/Drive Inverter/NMT Trasition Command/Undefined state ==
  Action Port : ActionPort  ActionPortLabel=case [ 1 2 8 ]:
  Bus Creator : BusCreator  Inputs=7
  Constant : Constant  Value=0  OutDataTypeStr=double
  Constant1 : Constant  Value=double(0)
  Constant2 : Constant  Value=boolean(0)
  Constant3 : Constant  Value=0  OutDataTypeStr=uint8
  Constant4 : Constant  Value=boolean(0)
  Constant5 : Constant  Value=uint8(0)
  Constant6 : Constant  Value=uint8(0)
  Header : Blocks_lib/Header  width=Portrait  addtext=''
  Cmd : Outport  VectorParamsAs1DForOutWhenUnconnected=off
  wires:
  Constant3/1 -> Bus Creator/1  "VCU1StateCmd [bool]"
  Constant/1 -> Bus Creator/2  "TrqCmd [Nm]"
  Constant1/1 -> Bus Creator/3  "SpdCmd [rpm]"
  Bus Creator/1 -> Cmd/1
  Constant2/1 -> Bus Creator/4  "VCU1_2_Transmit [bool]"
  Constant4/1 -> Bus Creator/5  "NMT_Xmit [bool]"
  Constant5/1 -> Bus Creator/6  "NMT_StateDmd"
  Constant6/1 -> Bus Creator/7  "NMT_Target_Node"

== system VCMGCM1962020b_v2/Fgnd/Actuators/CAN/Drive Inverter/State Transition Command1/Error ==
  Action Port : ActionPort
  Bus Creator : BusCreator  Inputs=4
  Constant : Constant  Value=0  OutDataTypeStr=double
  Constant1 : Constant  Value=double(0)
  Constant2 : Constant  Value=boolean(1)
  Constant3 : Constant  Value=2  OutDataTypeStr=uint8
  Header : Blocks_lib/Header  width=Portrait  addtext=''
  Cmd : Outport  VectorParamsAs1DForOutWhenUnconnected=off
  wires:
  Constant2/1 -> Bus Creator/4  "VCU1_2_Transmit [bool]"
  Bus Creator/1 -> Cmd/1
  Constant1/1 -> Bus Creator/3  "SpdCmd [rpm]"
  Constant/1 -> Bus Creator/2  "TrqCmd [Nm]"
  Constant3/1 -> Bus Creator/1  "AppCtrlCode [bool]"

== system VCMGCM1962020b_v2/Fgnd/Actuators/CAN/Drive Inverter/State Transition Command1/Init State ==
  Action Port : ActionPort
  Bus Creator : BusCreator  Inputs=4
  Constant : Constant  Value=0  OutDataTypeStr=double
  Constant2 : Constant  Value=boolean(0)
  Constant3 : Constant  Value=0  OutDataTypeStr=uint8
  Constant4 : Constant  Value=double(0)
  Header : Blocks_lib/Header  width=Portrait  addtext=''
  Cmd : Outport  VectorParamsAs1DForOutWhenUnconnected=off
  wires:
  Constant2/1 -> Bus Creator/4  "VCU1_2_Transmit [bool]"
  Bus Creator/1 -> Cmd/1
  Constant4/1 -> Bus Creator/3  "SpdCmd [rpm]"
  Constant/1 -> Bus Creator/2  "TrqCmd [Nm]"
  Constant3/1 -> Bus Creator/1  "AppCtrlCode [bool]"

== system VCMGCM1962020b_v2/Fgnd/Actuators/CAN/Drive Inverter/State Transition Command1/Off ==
  Input : Inport
  Action Port : ActionPort
  Bus Creator : BusCreator  Inputs=4
  Bus Selector : BusSelector  OutputSignals=Control.DrvInvtr.DrvInvtrEnblReq [Bool]
  Constant : Constant  Value=0  OutDataTypeStr=double
  Constant2 : Constant  Value=boolean(1)
  Constant3 : Constant  Value=0  OutDataTypeStr=uint8
  Constant4 : Constant  OutDataTypeStr=uint8
  Constant5 : Constant  Value=double(0)
  Header : Blocks_lib/Header  width=Portrait  addtext=''
  Multiport Switch : MultiPortSwitch  DataPortOrder=Zero-based contiguous  Inputs=2  zeroidx=on
  Cmd : Outport  VectorParamsAs1DForOutWhenUnconnected=off
  wires:
  Constant2/1 -> Bus Creator/4  "VCU1_2_Transmit [bool]"
  Bus Creator/1 -> Cmd/1
  Constant5/1 -> Bus Creator/3  "SpdCmd [rpm]"
  Constant/1 -> Bus Creator/2  "TrqCmd [Nm]"
  Input/1 -> Bus Selector/1
  Bus Selector/1 -> Multiport Switch/1  "<DrvInvtrEnblReq [Bool]>"
  Constant3/1 -> Multiport Switch/2
  Constant4/1 -> Multiport Switch/3
  Multiport Switch/1 -> Bus Creator/1  "AppCtrlCode [bool]"

== system VCMGCM1962020b_v2/Fgnd/Actuators/CAN/Drive Inverter/State Transition Command1/Run ==
  Input : Inport
  Action Port : ActionPort
  Bus Creator : BusCreator  Inputs=4
  Bus Selector1 : BusSelector  OutputSignals=Control.DrvInvtr.DrvInvtrEnblReq [Bool],Control.DrvInvtr.MtrTrqReq.DrvTrqReq.DrvTrqReqFinal [Nm]
  Constant1 : Constant  Value=double(0)
  Constant2 : Constant  Value=boolean(1)
  Constant4 : Constant  Value=0  OutDataTypeStr=uint8
  Constant5 : Constant  OutDataTypeStr=uint8
  Header : Blocks_lib/Header  width=Portrait  addtext=''
  Multiport Switch : MultiPortSwitch  DataPortOrder=Zero-based contiguous  Inputs=2  zeroidx=on
  Zero-Order Hold : ZeroOrderHold  SampleTime=-1
  Cmd : Outport  VectorParamsAs1DForOutWhenUnconnected=off
  wires:
  Constant2/1 -> Bus Creator/4  "VCU1_2_Transmit [bool]"
  Bus Creator/1 -> Cmd/1
  Constant1/1 -> Bus Creator/3  "SpdCmd [rpm]"
  Bus Selector1/2 -> Zero-Order Hold/1  "<DrvTrqReqFinal [Nm]>"
  Zero-Order Hold/1 -> Bus Creator/2  "TrqCmd [Nm]"
  Multiport Switch/1 -> Bus Creator/1  "AppCtrlCode [bool]"
  Constant5/1 -> Multiport Switch/3
  Constant4/1 -> Multiport Switch/2
  Input/1 -> Bus Selector1/1
  Bus Selector1/1 -> Multiport Switch/1  "<DrvInvtrEnblReq [Bool]>"

== system VCMGCM1962020b_v2/Fgnd/Actuators/CAN/Drive Inverter/State Transition Command1/Undefined state ==
  Action Port : ActionPort
  Bus Creator : BusCreator  Inputs=4
  Constant : Constant  Value=0  OutDataTypeStr=double
  Constant1 : Constant  Value=double(0)
  Constant2 : Constant  Value=boolean(0)
  Constant3 : Constant  Value=0  OutDataTypeStr=uint8
  Header : Blocks_lib/Header  width=Portrait  addtext=''
  Cmd : Outport  VectorParamsAs1DForOutWhenUnconnected=off
  wires:
  Constant3/1 -> Bus Creator/1  "AppCtrlCode [bool]"
  Constant/1 -> Bus Creator/2  "TrqCmd [Nm]"
  Constant1/1 -> Bus Creator/3  "SpdCmd [rpm]"
  Bus Creator/1 -> Cmd/1
  Constant2/1 -> Bus Creator/4  "VCU1_2_Transmit [bool]"

== system VCMGCM1962020b_v2/Fgnd/Actuators/CAN/Other/A//C Compressor/MsgName ==
  Data : Inport
  Bus Selector : BusSelector  OutputSignals=Control.Other.Other.SysWake [Bool]
  CANTxMsgEnbl : Blocks_lib/CANTxMsgEnbl  custom=on  custom_nam=[nam '---']  msgnam=ACCREQ
  Header : Blocks_lib/Header  width=Portrait  addtext=''
  MsgTx : Subsystem
  wires:
  Data/1 -> MsgTx/1(Data), Bus Selector/1
  Bus Selector/1 -> CANTxMsgEnbl/1  "<SysWake [Bool]>"
  CANTxMsgEnbl/1 -> MsgTx/Enable

== system VCMGCM1962020b_v2/Fgnd/Actuators/CAN/Other/Cooling Pump 1/MsgName ==
  Data : Inport
  Bus Selector : BusSelector  OutputSignals=Control.Other.Other.SysWake [Bool]
  CANTxMsgEnbl : Blocks_lib/CANTxMsgEnbl  custom=on  custom_nam=[nam '---']  msgnam=CoolPump1EAPMCPC
  Header : Blocks_lib/Header  width=Portrait  addtext=''
  MsgTx : Subsystem
  wires:
  CANTxMsgEnbl/1 -> MsgTx/Enable
  Bus Selector/1 -> CANTxMsgEnbl/1  "<SysWake [Bool]>"
  Data/1 -> Bus Selector/1, MsgTx/1(Data)

== system VCMGCM1962020b_v2/Fgnd/Actuators/CAN/Other/Cooling Pump 2/MsgName ==
  Data : Inport
  Bus Selector : BusSelector  OutputSignals=Control.Other.Other.SysWake [Bool]
  CANTxMsgEnbl : Blocks_lib/CANTxMsgEnbl  custom=on  custom_nam=[nam '---']  msgnam=CoolPump2EAPMCPC
  Header : Blocks_lib/Header  width=Portrait  addtext=''
  MsgTx : Subsystem
  wires:
  Data/1 -> MsgTx/1(Data), Bus Selector/1
  Bus Selector/1 -> CANTxMsgEnbl/1  "<SysWake [Bool]>"
  CANTxMsgEnbl/1 -> MsgTx/Enable

== system VCMGCM1962020b_v2/Fgnd/Actuators/CAN/Other/Heater/MsgName ==
  Data : Inport
  Bus Selector : BusSelector  OutputSignals=Control.Other.Other.SysWake [Bool]
  CANTxMsgEnbl : Blocks_lib/CANTxMsgEnbl  custom=off  custom_nam='---'  msgnam=Data_Set_1
  Header : Blocks_lib/Header  width=Portrait  addtext=''
  MsgTx : Subsystem
  wires:
  CANTxMsgEnbl/1 -> MsgTx/Enable
  Bus Selector/1 -> CANTxMsgEnbl/1  "<SysWake [Bool]>"
  Data/1 -> Bus Selector/1, MsgTx/1(Data)

== system VCMGCM1962020b_v2/Fgnd/Actuators/CAN/Other/MPDM/MsgName ==
  Data : Inport
  Bus Selector : BusSelector  OutputSignals=Control.Other.Other.MPDMWake [Bool]
  CANTxMsgEnbl : Blocks_lib/CANTxMsgEnbl  custom=on  custom_nam=[nam '---']  msgnam=MPDMRelayCommand
  Header : Blocks_lib/Header  width=Portrait  addtext=''
  MsgTx : Subsystem
  wires:
  CANTxMsgEnbl/1 -> MsgTx/Enable
  Bus Selector/1 -> CANTxMsgEnbl/1  "<MPDMWake [Bool]>"
  Data/1 -> Bus Selector/1, MsgTx/1(Data)

== system VCMGCM1962020b_v2/Fgnd/Actuators/CAN/Other/Power Steering Pump Inverter/MsgName ==
  Data : Inport
  Bus Selector : BusSelector  OutputSignals=Control.Other.Other.SysWake [Bool]
  CANTxMsgEnbl : Blocks_lib/CANTxMsgEnbl  custom=on  custom_nam=[nam '---']  msgnam=PSPInvtrHC2_Demands
  Header : Blocks_lib/Header  width=Portrait  addtext=''
  MsgTx : Subsystem
  wires:
  CANTxMsgEnbl/1 -> MsgTx/Enable
  Bus Selector/1 -> CANTxMsgEnbl/1  "<SysWake [Bool]>"
  Data/1 -> Bus Selector/1, MsgTx/1(Data)

== system VCMGCM1962020b_v2/Fgnd/Actuators/CAN/Other/Power Steering Pump Inverter/PSPInvtrHC1_Demands ==
  Data : Inport
  Bus Selector : BusSelector  OutputSignals=Control.Other.Other.SysWake [Bool]
  CANTxMsgEnbl : Blocks_lib/CANTxMsgEnbl  custom=on  custom_nam=[nam '---']  msgnam=PSPInvtrHC1_Demands
  Header : Blocks_lib/Header  width=Portrait  addtext=''
  MsgTx : Subsystem
  wires:
  CANTxMsgEnbl/1 -> MsgTx/Enable
  Bus Selector/1 -> CANTxMsgEnbl/1  "<SysWake [Bool]>"
  Data/1 -> Bus Selector/1, MsgTx/1(Data)

== system VCMGCM1962020b_v2/Fgnd/Actuators/CAN/Other/Power Steering Pump Inverter/PSPInvtrHC3_Battery_Demands ==
  Data : Inport
  Bus Selector : BusSelector  OutputSignals=Control.Other.Other.SysWake [Bool]
  CANTxMsgEnbl : Blocks_lib/CANTxMsgEnbl  custom=on  custom_nam=[nam '---']  msgnam=PSPInvtrHC3_Battery_Demands
  Header : Blocks_lib/Header  width=Portrait  addtext=''
  MsgTx : Subsystem
  wires:
  CANTxMsgEnbl/1 -> MsgTx/Enable
  Bus Selector/1 -> CANTxMsgEnbl/1  "<SysWake [Bool]>"
  Data/1 -> Bus Selector/1, MsgTx/1(Data)

== system VCMGCM1962020b_v2/Fgnd/Control/Drive Inverter/Motor Torque Request/Current//Torque Split/Inverter Current Limits ==
  Data : Inport
  Add : Sum  Inputs=+-  InputSameDT=on  OutDataTypeStr=Inherit: Same as first input
  Add1 : Sum  InputSameDT=on  OutDataTypeStr=Inherit: Same as first input
  Bus Selector : BusSelector  OutputSignals=VirtualSensors.Batt.BattDCL [A],VirtualSensors.PDU.HVAccCur [A]
  Bus Selector1 : BusSelector  OutputSignals=VirtualSensors.Batt.BattCCL [A],VirtualSensors.PDU.HVAccCur [A]
  Header : Blocks_lib/Header  width=Portrait  addtext=''
  Saturation : Saturate  UpperLimit=inf  LowerLimit=0
  MCL : Outport  VectorParamsAs1DForOutWhenUnconnected=off
  GCL : Outport  Port=2  VectorParamsAs1DForOutWhenUnconnected=off
  wires:
  Bus Selector1/2 -> Add1/2  "<HVAccCur [A]>"
  Bus Selector/2 -> Add/2  "<HVAccCur [A]>"
  Bus Selector1/1 -> Add1/1  "<BattCCL [A]>"
  Add/1 -> Saturation/1
  Bus Selector/1 -> Add/1  "<BattDCL [A]>"
  Add1/1 -> GCL/1
  Saturation/1 -> MCL/1
  Data/1 -> Bus Selector1/1, Bus Selector/1

== system VCMGCM1962020b_v2/Fgnd/Control/Drive Inverter/Motor Torque Request/Driver Torque Request/Cruise Control ==
  Data : Inport
  DrvTrq : Inport  Port=2
  Bus Creator : BusCreator  Inputs=2
  Bus Selector : BusSelector  OutputSignals=CCActv [Bool]
  Control : Subsystem
  Header : Blocks_lib/Header  width=Portrait  addtext=''
  Multiport Switch : MultiPortSwitch  DataPortOrder=Zero-based contiguous  Inputs=2  zeroidx=on
  Setpoint : Subsystem
  CC : Outport  VectorParamsAs1DForOutWhenUnconnected=off
  Nm : Outport  Port=2  VectorParamsAs1DForOutWhenUnconnected=off
  wires:
  Control/1(Nm) -> Bus Creator/2, Multiport Switch/3  "CCTrqReq [Nm]"
  Data/1 -> Setpoint/1(Data), Control/1(Data)
  Setpoint/1(Setpt) -> Control/3(Setpt), Bus Selector/1, Bus Creator/1
  Bus Creator/1 -> CC/1  "CC"
  Bus Selector/1 -> Control/Enable, Multiport Switch/1  "<CCActv [Bool]>"
  Multiport Switch/1 -> Nm/1
  DrvTrq/1 -> Control/2(PedTrq), Multiport Switch/2

== system VCMGCM1962020b_v2/Fgnd/Control/Drive Inverter/Motor Torque Request/Driver Torque Request/Driveability ==
  Data : Inport
  DrvTrq : Inport  Port=2
  Filt : Blocks_lib/Filt  nam='DrvTrqReqFiltTC'  group=group  samptime=samptime
  Header : Blocks_lib/Header  width=Portrait  addtext=''
  Rate Limit : Subsystem
  RateLim : Blocks_lib/RateLim  samptime=samptime
  Unit Delay : UnitDelay  SampleTime=-1  HasFrameUpgradeWarning=on
  raptor_measurement : Raptor_lib/Data Storage/raptor_measurement  paramName='DrvTrqReqFinal'  nameSource=Parameter  calDispType=Number  calEnum={'Disabled', 'Enabled'}  calGain=1  calOffset=0  calMax=inf  calMin=-inf  calFormat=''  calUnit='Nm'  calHelp='Driver torque request (final)'  calAccess=1  calFunction=group  calVisible=on
      settings: SourceProductName=Raptor
  Nm : Outport  VectorParamsAs1DForOutWhenUnconnected=off
  wires:
  Unit Delay/1 -> Rate Limit/2(TrqReq)
  Data/1 -> Rate Limit/1(Data)
  Filt/1 -> RateLim/1
  DrvTrq/1 -> Filt/1
  Rate Limit/1(Nm/s) -> RateLim/2
  RateLim/1 -> Nm/1, Unit Delay/1, raptor_measurement/1

== system VCMGCM1962020b_v2/Fgnd/Control/Drive Inverter/Motor Torque Request/Driver Torque Request/Pedal Torque Request ==
  Data : Inport
  APP When Two Pedal Driving : Subsystem
  Add : Sum  InputSameDT=on  OutDataTypeStr=Inherit: Same as first input
  Apply Sign to Vehicle Speed : Subsystem
  Bus Selector1 : BusSelector  OutputSignals=Control.Mode.PRNDMode [enum]
  CmprTo : Blocks_lib/CmprTo  op===  val='Rev'  enum=EnumLst.PRNDMode
  Creep Torque : Subsystem
  Gain : Gain  Gain=-1
  Header : Blocks_lib/Header  width=Portrait  addtext=''
  Meas&Ovrd : Blocks_lib/Meas&Ovrd  nam='DrvTrqReqRaw'  name_source=Parameter  view_as=Number  enum_struct={}  gain=1  min=-inf  max=inf  precision=''  units='Nm'  help='Driver torque request (raw)'  group=group
  Multiport Switch : MultiPortSwitch  DataPortOrder=Zero-based contiguous  Inputs=2  zeroidx=on
  raptor_table_2d : Raptor_lib/Table Lookup/raptor_table_2d  dataName='APPTrqReqMap'  initValue=zeros(21,11)  dataType=double  storage=Calibration  initValueX=[1:11]  initValueY=[1:21]  dataTypeXY=double  storageXY=Calibration  calVisible=on  showTable=on  calGain=1.0  calOffset=0.0  calMax=Inf  calMin=-Inf  calFormat='-1'  calUnit='Nm'  calHelp='APP-based torque request'  showBreakpointX=on  dataNameX='APP11IdxArr'  calGainX=1.0  calOffsetX=0.0  calMaxX=Inf  calMinX=-Inf  calFormatX='-1'  calUnitX='%'  calHelpX='Index array'  showBreakpointY=on  dataNameY='VehSpd21IdxArr'  calGainY=1.0  calOffsetY=0.0  calMaxY=Inf  calMinY=-Inf  calFormatY='-1'  calUnitY='kph'  calHelpY='Index array'  calAccess=1  calFunction=group  measureEnable=on  mName='APPTrqReq'
      settings: SourceProductName=Raptor
  Nm : Outport  VectorParamsAs1DForOutWhenUnconnected=off
  wires:
  Meas&Ovrd/1 -> Nm/1
  Creep Torque/1(Nm) -> Add/2
  raptor_table_2d/1 -> Add/1
  Multiport Switch/1 -> Meas&Ovrd/1
  Bus Selector1/1 -> CmprTo/1  "<PRNDMode [enum]>"
  CmprTo/1 -> Multiport Switch/1
  Gain/1 -> Multiport Switch/3
  Data/1 -> Bus Selector1/1, APP When Two Pedal Driving/1(Data), Creep Torque/1(Data), Apply Sign to Vehicle Speed/1(Data)
  Apply Sign to Vehicle Speed/1(kph) -> raptor_table_2d/1
  Add/1 -> Gain/1, Multiport Switch/2
  APP When Two Pedal Driving/1(%) -> raptor_table_2d/2

== system VCMGCM1962020b_v2/Fgnd/Control/Drive Inverter/Motor Torque Request/Driver Torque Request/Vehicle Speed Limiter ==
  note: Note: Only apply vehicle speed limit multiplier
      | if vehicle is moving in desired direction.
  Data : Inport
  DrvTrq : Inport  Port=2
  Add : Sum  Inputs=+-
  Bus Selector : BusSelector  OutputSignals=VirtualSensors.Spd.VehSpd [kph]
  Bus Selector1 : BusSelector  OutputSignals=VirtualSensors.Spd.VehDir [enum],Control.Mode.PRNDMode [enum]
  CmprTo : Blocks_lib/CmprTo  op===  val='Fwd'  enum=EnumLst.VehDir
  CmprTo1 : Blocks_lib/CmprTo  op===  val='Drv'  enum=EnumLst.PRNDMode
  CmprTo2 : Blocks_lib/CmprTo  op===  val='Rev'  enum=EnumLst.VehDir
  CmprTo3 : Blocks_lib/CmprTo  op===  val='Rev'  enum=EnumLst.PRNDMode
  Header : Blocks_lib/Header  width=Portrait  addtext=''
  Logical Operator2 : Logic  Operator=OR  OutDataTypeStr=boolean
  Logical Operator4 : Logic  OutDataTypeStr=boolean
  Logical Operator5 : Logic  OutDataTypeStr=boolean
  Multiport Switch : MultiPortSwitch  DataPortOrder=Zero-based contiguous  Inputs=2  zeroidx=on
  Product : Product
  Vehicle Speed Limit : Subsystem
  raptor_measurement : Raptor_lib/Data Storage/raptor_measurement  paramName='DrvTrqReqVehSpdLim'  nameSource=Parameter  calDispType=Number  calEnum={'Disabled', 'Enabled'}  calGain=1  calOffset=0  calMax=inf  calMin=-inf  calFormat=''  calUnit='Nm'  calHelp='Driver torque request (after vehicle speed limit multiplier applied)'  calAccess=1  calFunction=group  calVisible=on
      settings: SourceProductName=Raptor
  raptor_table_1d : Raptor_lib/Table Lookup/raptor_table_1d  dataName='DrvTrqReqMultpVehSpdHiTbl'  initValue=zeros(1,7)  dataType=double  storage=Calibration  initValueX=[1:7]  dataTypeXY=double  storageXY=Calibration  calVisible=on  showTable=on  calGain=1.0  calOffset=0.0  calMax=Inf  calMin=-Inf  calFormat='-1'  calUnit='multp'  calHelp='Driver torque request multiplier (at high vehicle speed)'  showBreakpoint=on  dataNameX='VehSpdHiDelta07IdxArr'  calGainX=1.0  calOffsetX=0.0  calMaxX=Inf  calMinX=-Inf  calFormatX='-1'  calUnitX='kph'  calHelpX='Index array'  calAccess=1  calFunction=group  measureEnable=on  mName='DrvTrqReqMultpVehSpdHi'
      settings: SourceProductName=Raptor
  kph : Outport  VectorParamsAs1DForOutWhenUnconnected=off
  Nm : Outport  Port=2  VectorParamsAs1DForOutWhenUnconnected=off
  wires:
  Vehicle Speed Limit/1(kph) -> kph/1, Add/2
  Bus Selector1/2 -> CmprTo1/1, CmprTo3/1  "<PRNDMode [enum]>"
  Bus Selector1/1 -> CmprTo/1, CmprTo2/1  "<VehDir [enum]>"
  DrvTrq/1 -> Multiport Switch/2, Product/1
  Multiport Switch/1 -> Nm/1, raptor_measurement/1
  Product/1 -> Multiport Switch/3
  CmprTo3/1 -> Logical Operator5/2
  CmprTo1/1 -> Logical Operator4/2
  Logical Operator2/1 -> Multiport Switch/1
  CmprTo/1 -> Logical Operator4/1
  Logical Operator4/1 -> Logical Operator2/1
  CmprTo2/1 -> Logical Operator5/1
  Logical Operator5/1 -> Logical Operator2/2
  Data/1 -> Bus Selector/1, Bus Selector1/1
  Add/1 -> raptor_table_1d/1
  Bus Selector/1 -> Add/1  "<VehSpd [kph]>"
  raptor_table_1d/1 -> Product/2
